simulink model "L3"  (R2015a)
settings: Solver=ode3  SolverMode=SingleTasking  StartTime=0.0  StopTime=50  FixedStep=1e-3  RelTol=1e-3
undefined symbols (not defined in the file or in its folder): magnitude
settings Model: CovMetricSettings=dwe  CovHtmlReporting=off  covSaveCumulativeToWorkspaceVar=off  CovSaveSingleToWorkspaceVar=off  CovExternalEMLEnable=on  Creator=Daniel  LastModifiedBy=Daniel
settings DataIOCC: LimitDataPoints=off  SaveFormat=Dataset
settings DebuggingCC: SFUnexpectedBacktrackingDiag=error  SFNoUnconditionalDefaultTransitionDiag=error
settings HardwareCC: ProdBitPerPointer=64  ProdLargestAtomicFloat=Float  ProdIntDivRoundTo=Zero  ProdEndianess=LittleEndian  ProdHWDeviceType=Specified
settings ModelReferenceCC: PropagateSignalLabelsOutOfModel=on
settings GRTTargetCC: TargetLangStandard=C99 (ISO)  GeneratePreprocessorConditionals=Use local settings

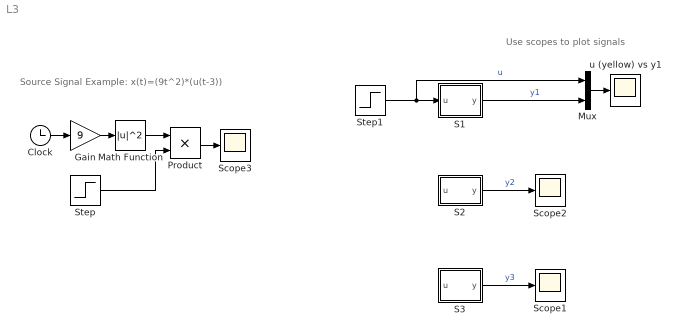
== system L3 ==
  note: Use scopes to plot signals
  note: Source Signal Example: x(t)=(9t^2)*(u(t-3))
  Clock : Clock
  Gain : Gain  Gain=9
  Math Function : Math  Operator=magnitude^2  SaturateOnIntegerOverflow=on
  Mux : Mux  Inputs=2
  Product : Product
  S1 : Subsystem
  S2 : Subsystem
  S3 : Subsystem
  Scope1 : Scope
      settings: YMin=-1.00000  YMax=1.00000
  Scope2 : Scope
      settings: YMin=-5.76618  YMax=51.89562  SaveName=ScopeData2
  Scope3 : Scope
      settings: YMin=-1.00000  YMax=1.00000  SaveName=ScopeData3
  Step : Step  Time=3  SampleTime=0
  Step1 : Step  Time=0  SampleTime=0
  u (yellow) vs y1 : Scope
      settings: YMin=-1.00000  YMax=1.00000
  wires:
  S2/1(y) -> Scope2/1  "y2"
  S3/1(y) -> Scope1/1  "y3"
  Gain/1 -> Math Function/1
  Math Function/1 -> Product/1
  Product/1 -> Scope3/1
  Clock/1 -> Gain/1
  Step/1 -> Product/2
  Mux/1 -> u (yellow) vs y1/1
  S1/1(y) -> Mux/2  "y1"
  Step1/1 -> Mux/1, S1/1(u)  "u"

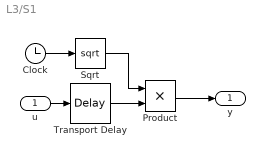
== system L3/S1 ==
  u : Inport
  Clock : Clock
  Product : Product
  Sqrt : Sqrt  SaturateOnIntegerOverflow=on
  Transport Delay : TransportDelay
  y : Outport
  wires:
  Transport Delay/1 -> Product/2
  Clock/1 -> Sqrt/1
  u/1 -> Transport Delay/1
  Product/1 -> y/1
  Sqrt/1 -> Product/1

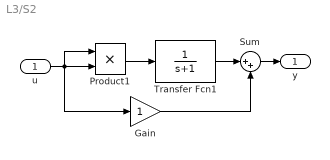
== system L3/S2 ==
  u : Inport
  Gain : Gain
  Product1 : Product
  Sum : Sum  Inputs=|++
  Transfer Fcn1 : TransferFcn  Denominator=[1 1]
  y : Outport
  wires:
  Sum/1 -> y/1
  u/1 -> Gain/1, Product1/1, Product1/2
  Product1/1 -> Transfer Fcn1/1
  Transfer Fcn1/1 -> Sum/1
  Gain/1 -> Sum/2

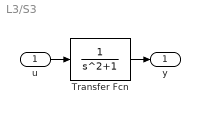
== system L3/S3 ==
  u : Inport
  Transfer Fcn : TransferFcn  Denominator=[1 0 1]
  y : Outport
  wires:
  Transfer Fcn/1 -> y/1
  u/1 -> Transfer Fcn/1
